simulink model "testing_library"  (R2020b)
settings: Solver=VariableStepAuto  StartTime=0.0  StopTime=inf  RelTol=1e-3
libraries: DSX_Lib x3
settings Model: Creator=16047  LastModifiedBy=16047

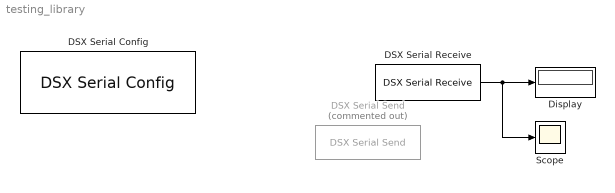
== system testing_library ==
  DSX Serial Config : DSX_Lib/DSX Serial Config  BaudRate=115200
      settings: SourceProductName=DSX Library
  DSX Serial Receive : DSX_Lib/Serial Blocks/DSX Serial Receive  sike=sike
      settings: SourceProductName=DSX Library
  DSX Serial Send : DSX_Lib/Serial Blocks/DSX Serial Send  Commented=on  data=balls
      settings: SourceProductName=DSX Library
  Display : Display
      settings: Decimation=25
  Scope : Scope
  wires:
  DSX Serial Receive/1 -> Scope/1, Display/1
